simulink model "HardwareModel"  (R2023a)
settings: Solver=ode4  StartTime=0.0  StopTime=inf  FixedStep=Parameters.Simulink.time_step_s  RelTol=1e-3
undefined symbols (not defined in the file or in its folder): flight_mode, FLIGHT_MODE, joystick, Parameters, wait_time_s
libraries: px4lib x121, matrix_library x9, px4uORBlib x3, sharedutil x2, simulink_extras x1, vrlib x1
settings Model: ExtModeTrigDuration=10  Creator=thesa  LastModifiedBy=thesa
settings SolverCC: PositivePriorityOrder=on
settings OptimizationCC: EnhancedBackFolding=on  PassReuseOutputArgsAs=Individual arguments  ZeroExternalMemoryAtStartup=off  ZeroInternalMemoryAtStartup=off  MaxStackSize=64  OptimizeBlockOrder=speed  DifferentSizesBufferReuse=on  OptimizationCustomize=off  EfficientTunableParamExpr=on
settings DebuggingCC: ParameterTunabilityLossMsg=error
settings HardwareCC: ProdBitPerPointer=32  ProdBitPerSizeT=32  ProdBitPerPtrDiffT=32  ProdLargestAtomicInteger=Long  ProdLargestAtomicFloat=Double  ProdWordSize=32  ProdLongLongMode=on  ProdHWDeviceType=ARM Compatible->ARM Cortex
settings SFSimCC: SimTargetLang=C++
settings RTWCC: Description=Embedded Coder  SystemTargetFile=ert.tlc  HardwareBoard=PX4 Cube Orange  TLCOptions="-aInlineSetEventsForThisBaseRateFcn=TLC_FALSE -aSuppressMultiTaskScheduler=TLC_FALSE  -aRateBasedStepFcn=0"  TemplateMakefile=ert_default_tmf  Toolchain=GNU Tools for PX4 Autopilots  TargetLang=C++
settings CodeAppCC: ForceParamTrailComments=on  IgnoreCustomStorageClasses=off  OperatorAnnotations=on  SimulinkDataObjDesc=on  SFDataObjDesc=on  InsertBlockDesc=on
settings ERTTargetCC: SupportVariableSizeSignals=on  ExtModeTransport=3  ExtModeStaticAlloc=on  ExtModeStaticAllocSize=1024  ExtModeMexFile=ext_xcp  ExtModeIntrfLevel=Level2 - Open

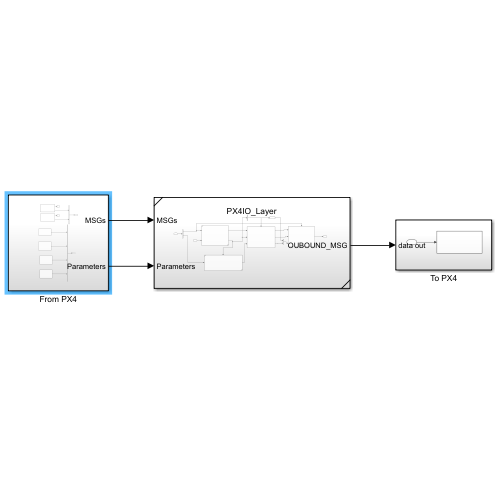
[thumbnail: Simulink's stored preview of the top-level diagram]
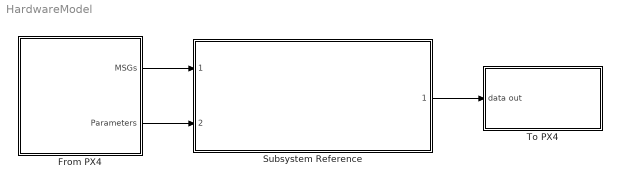
== system HardwareModel ==
  From PX4 : Subsystem
  Subsystem Reference : Subsystem  ReferencedSubsystem=PX4IO_Layer
  To PX4 : Subsystem
  wires:
  From PX4/1(MSGs) -> Subsystem Reference/1
  Subsystem Reference/1 -> To PX4/1(data out)
  From PX4/2(Parameters) -> Subsystem Reference/2

== system HardwareModel/From PX4 ==
  Bus Creator : BusCreator  Inputs=4
  Bus Creator1 : BusCreator  Inputs=2
  PX4 uORB Read : px4uORBlib/PX4 uORB Read  uORBTopic=debug_array  selectInstance=simulink_inbound  SampleTime=-1  BlockingMode=off  BlockTimeout=1e-3
  PX4 uORB Read1 : px4uORBlib/PX4 uORB Read  uORBTopic=debug_array  selectInstance=simulink_guidance  SampleTime=-1  BlockingMode=off  BlockTimeout=1e-3
  Subsystem1 : Subsystem
  Subsystem2 : Subsystem
  Subsystem3 : Subsystem
  Subsystem5 : Subsystem
  Terminator : Terminator
  Terminator1 : Terminator
  MSGs : Outport
  Parameters : Outport  Port=2
  wires:
  PX4 uORB Read/1 -> Terminator/1
  PX4 uORB Read/2 -> Bus Creator1/1  "INBOUND_MSG"
  Subsystem2/1(Control Gains) -> Bus Creator/2  "Control Gains"
  Subsystem3/1(Vehicle Parameters) -> Bus Creator/1  "Vehicle Parameters"
  Subsystem5/1(Pilot Input) -> Bus Creator/4  "Pilot Input"
  Bus Creator1/1 -> MSGs/1
  PX4 uORB Read1/1 -> Terminator1/1
  PX4 uORB Read1/2 -> Bus Creator1/2  "GUIDANCE_MSG"
  Subsystem1/1(Control Logic) -> Bus Creator/3  "Control Logic"
  Bus Creator/1 -> Parameters/1

== system HardwareModel/To PX4 ==
  data out : Inport
  PX4 uORB Write1 : px4uORBlib/PX4 uORB Write  uORBTopic=debug_array  selectInstance=simulink_outbound  MessageQueueLen=1
  wires:
  data out/1 -> PX4 uORB Write1/1

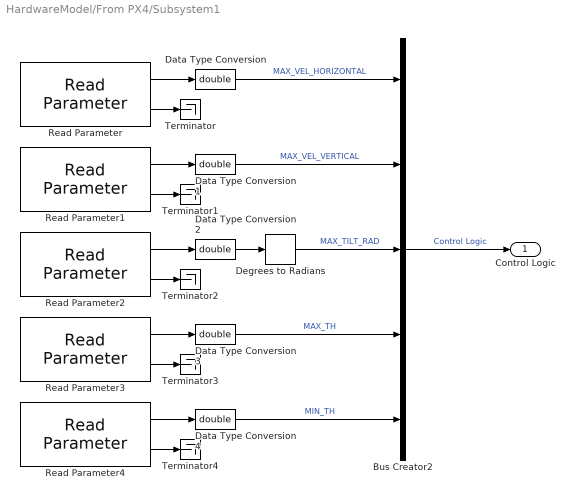
== system HardwareModel/From PX4/Subsystem1 ==
  Bus Creator2 : BusCreator  Inputs=5
  Data Type Conversion{,1..4} (5 alike) : DataTypeConversion  OutDataTypeStr=double  SaturateOnIntegerOverflow=off  RndMeth=Floor
  Degrees to Radians : simulink_extras/Transformations/Degrees to Radians
  Read Parameter : px4lib/Read Parameter  ParameterName=SM_MAX_VEL_HOR  DataType=FLOAT  SampleTime=-1
  Read Parameter1 : px4lib/Read Parameter  ParameterName=SM_MAX_VEL_VER  DataType=FLOAT  SampleTime=-1
  Read Parameter2 : px4lib/Read Parameter  ParameterName=SM_MAX_TILT  DataType=FLOAT  SampleTime=-1
  Read Parameter3 : px4lib/Read Parameter  ParameterName=SM_MAX_TH  DataType=FLOAT  SampleTime=-1
  Read Parameter4 : px4lib/Read Parameter  ParameterName=SM_MIN_TH  DataType=FLOAT  SampleTime=-1
  Terminator{,1..4} (5 alike) : Terminator
  Control Logic : Outport
  wires:
  Read Parameter4/1 -> Data Type Conversion4/1
  Read Parameter3/1 -> Data Type Conversion3/1
  Read Parameter1/1 -> Data Type Conversion1/1
  Bus Creator2/1 -> Control Logic/1  "Control Logic"
  Read Parameter/1 -> Data Type Conversion/1
  Read Parameter2/1 -> Data Type Conversion2/1
  Degrees to Radians/1 -> Bus Creator2/3  "MAX_TILT_RAD"
  Read Parameter/2 -> Terminator/1
  Read Parameter1/2 -> Terminator1/1
  Read Parameter3/2 -> Terminator3/1
  Read Parameter2/2 -> Terminator2/1
  Read Parameter4/2 -> Terminator4/1
  Data Type Conversion/1 -> Bus Creator2/1  "MAX_VEL_HORIZONTAL"
  Data Type Conversion1/1 -> Bus Creator2/2  "MAX_VEL_VERTICAL"
  Data Type Conversion2/1 -> Degrees to Radians/1
  Data Type Conversion3/1 -> Bus Creator2/4  "MAX_TH"
  Data Type Conversion4/1 -> Bus Creator2/5  "MIN_TH"

== system HardwareModel/From PX4/Subsystem2 ==
  " K-matrix control (LQR, H-inf, etc.)" : Subsystem
  Bus Creator2 : BusCreator  Inputs=9
  Subsystem : Subsystem
  Subsystem1 : Subsystem
  Subsystem2 : Subsystem
  Subsystem3 : Subsystem
  Subsystem4 : Subsystem
  Subsystem5 : Subsystem
  Subsystem6 : Subsystem
  Subsystem7 : Subsystem
  Control Gains : Outport
  wires:
  Subsystem2/1(VEL_P) -> Bus Creator2/3  "K_vel"
  Subsystem/1(POS_P) -> Bus Creator2/1  "K_pos"
  Subsystem5/1(RATE_P) -> Bus Creator2/6  "K_omega"
  Bus Creator2/1 -> Control Gains/1  "Control Gains"
  Subsystem1/1(POS_I) -> Bus Creator2/2  "K_pos_int"
  Subsystem3/1(ACC_P) -> Bus Creator2/4  "K_acc"
  Subsystem4/1(ATT_P) -> Bus Creator2/5  "K_att"
  " K-matrix control (LQR, H-inf, etc.)"/1(K_matrix_control) -> Bus Creator2/9  "K_matrix_control"
  Subsystem6/1(RATE_I) -> Bus Creator2/7  "K_omega_I"
  Subsystem7/1(RATE_D) -> Bus Creator2/8  "K_omega_dot"

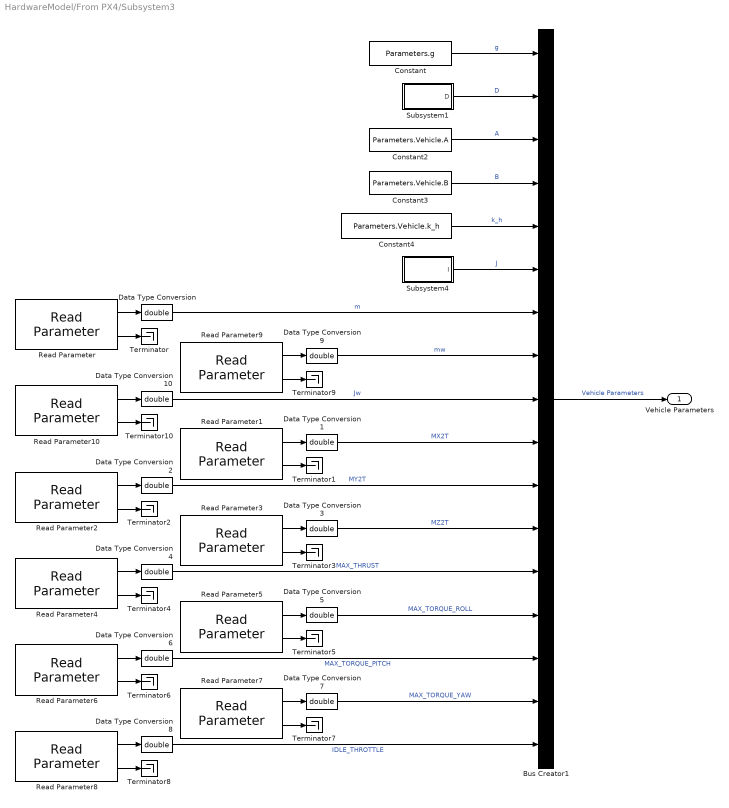
== system HardwareModel/From PX4/Subsystem3 ==
  Bus Creator1 : BusCreator  Inputs=17
  Constant : Constant  Value=Parameters.g
  Constant2 : Constant  Value=Parameters.Vehicle.A
  Constant3 : Constant  Value=Parameters.Vehicle.B
  Constant4 : Constant  Value=Parameters.Vehicle.k_h
  Data Type Conversion{,1..10} (11 alike) : DataTypeConversion  OutDataTypeStr=double  SaturateOnIntegerOverflow=off  RndMeth=Floor
  Read Parameter : px4lib/Read Parameter  ParameterName=SM_MASS  DataType=FLOAT  SampleTime=-1
  Read Parameter1 : px4lib/Read Parameter  ParameterName=SM_MX2T  DataType=FLOAT  SampleTime=-1
  Read Parameter10 : px4lib/Read Parameter  ParameterName=SM_I_ROTOR  DataType=FLOAT  SampleTime=-1
  Read Parameter2 : px4lib/Read Parameter  ParameterName=SM_MY2T  DataType=FLOAT  SampleTime=-1
  Read Parameter3 : px4lib/Read Parameter  ParameterName=SM_MZ2T  DataType=FLOAT  SampleTime=-1
  Read Parameter4 : px4lib/Read Parameter  ParameterName=SM_MAX_THRUST  DataType=FLOAT  SampleTime=-1
  Read Parameter5 : px4lib/Read Parameter  ParameterName=SM_MAX_MROLL  DataType=FLOAT  SampleTime=-1
  Read Parameter6 : px4lib/Read Parameter  ParameterName=SM_MAX_MPITCH  DataType=FLOAT  SampleTime=-1
  Read Parameter7 : px4lib/Read Parameter  ParameterName=SM_MAX_MYAW  DataType=FLOAT  SampleTime=-1
  Read Parameter8 : px4lib/Read Parameter  ParameterName=SM_IDLE_TH  DataType=FLOAT  SampleTime=-1
  Read Parameter9 : px4lib/Read Parameter  ParameterName=SM_MASS_ROTOR  DataType=FLOAT  SampleTime=-1
  Subsystem1 : Subsystem
  Subsystem4 : Subsystem
  Terminator{,1..10} (11 alike) : Terminator
  Vehicle Parameters : Outport
  wires:
  Subsystem4/1(I) -> Bus Creator1/6  "J"
  Constant3/1 -> Bus Creator1/4  "B"
  Constant/1 -> Bus Creator1/1  "g"
  Subsystem1/1(D) -> Bus Creator1/2  "D"
  Constant2/1 -> Bus Creator1/3  "A"
  Constant4/1 -> Bus Creator1/5  "k_h"
  Bus Creator1/1 -> Vehicle Parameters/1  "Vehicle Parameters"
  Data Type Conversion/1 -> Bus Creator1/7  "m"
  Data Type Conversion9/1 -> Bus Creator1/8  "mw"
  Data Type Conversion10/1 -> Bus Creator1/9  "Jw"
  Data Type Conversion1/1 -> Bus Creator1/10  "MX2T"
  Data Type Conversion2/1 -> Bus Creator1/11  "MY2T"
  Data Type Conversion3/1 -> Bus Creator1/12  "MZ2T"
  Data Type Conversion4/1 -> Bus Creator1/13  "MAX_THRUST"
  Data Type Conversion5/1 -> Bus Creator1/14  "MAX_TORQUE_ROLL"
  Data Type Conversion6/1 -> Bus Creator1/15  "MAX_TORQUE_PITCH"
  Data Type Conversion7/1 -> Bus Creator1/16  "MAX_TORQUE_YAW"
  Data Type Conversion8/1 -> Bus Creator1/17  "IDLE_THROTTLE"
  Read Parameter/2 -> Terminator/1
  Read Parameter/1 -> Data Type Conversion/1
  Read Parameter1/2 -> Terminator1/1
  Read Parameter1/1 -> Data Type Conversion1/1
  Read Parameter2/2 -> Terminator2/1
  Read Parameter2/1 -> Data Type Conversion2/1
  Read Parameter3/2 -> Terminator3/1
  Read Parameter3/1 -> Data Type Conversion3/1
  Read Parameter4/2 -> Terminator4/1
  Read Parameter4/1 -> Data Type Conversion4/1
  Read Parameter5/2 -> Terminator5/1
  Read Parameter5/1 -> Data Type Conversion5/1
  Read Parameter6/2 -> Terminator6/1
  Read Parameter6/1 -> Data Type Conversion6/1
  Read Parameter7/1 -> Data Type Conversion7/1
  Read Parameter7/2 -> Terminator7/1
  Read Parameter8/1 -> Data Type Conversion8/1
  Read Parameter8/2 -> Terminator8/1
  Read Parameter9/1 -> Data Type Conversion9/1
  Read Parameter9/2 -> Terminator9/1
  Read Parameter10/1 -> Data Type Conversion10/1
  Read Parameter10/2 -> Terminator10/1

== system HardwareModel/From PX4/Subsystem5 ==
  Bus Creator4 : BusCreator  Inputs=4
  Subsystem : Subsystem
  Subsystem1 : Subsystem
  Pilot Input : Outport
  wires:
  Subsystem/1(sticks) -> Bus Creator4/1  "Sticks"
  Bus Creator4/1 -> Pilot Input/1  "Pilot Input"
  Subsystem1/1(Parameters) -> Bus Creator4/4  "Parameters"
  Subsystem/2(FLIGHT_MODE) -> Bus Creator4/2  "FLIGHT_MODE"
  Subsystem/3(ARMED) -> Bus Creator4/3  "ARMED"

== system HardwareModel/From PX4/Subsystem2/ K-matrix control (LQR, H-inf, etc.) ==
  Bus Creator : BusCreator  Inputs=3
  Data Type Conversion9 : DataTypeConversion  OutDataTypeStr=boolean  SaturateOnIntegerOverflow=off  RndMeth=Floor
  Read Parameter9 : px4lib/Read Parameter  ParameterName=SM_EN_K_CONROL  DataType=INT32  SampleTime=-1
  Subsystem5 : Subsystem
  Subsystem6 : Subsystem
  Terminator9 : Terminator
  K_matrix_control : Outport
  wires:
  Bus Creator/1 -> K_matrix_control/1  "K_matrix_control"
  Subsystem6/1(K_matrix) -> Bus Creator/2  "K"
  Data Type Conversion9/1 -> Bus Creator/1  "EN"
  Subsystem5/1(K_pos_int) -> Bus Creator/3  "K_pos_int"
  Read Parameter9/2 -> Terminator9/1
  Read Parameter9/1 -> Data Type Conversion9/1

== system HardwareModel/From PX4/Subsystem2/Subsystem ==
  Create Diagonal Matrix : matrix_library/Create Diagonal Matrix
      settings: LibrarySourceBlock=|
      | simulink/Matrix
      | Operations/Create Diagonal
      | Matrix
  Data Type Conversion : DataTypeConversion  OutDataTypeStr=double  SaturateOnIntegerOverflow=off  RndMeth=Floor
  Mux : Mux  Inputs=3
  Read Parameter : px4lib/Read Parameter  ParameterName=SM_POS_P1  DataType=FLOAT  SampleTime=-1
  Read Parameter1 : px4lib/Read Parameter  ParameterName=SM_POS_P2  DataType=FLOAT  SampleTime=-1
  Read Parameter2 : px4lib/Read Parameter  ParameterName=SM_POS_P3  DataType=FLOAT  SampleTime=-1
  Terminator : Terminator
  Terminator1 : Terminator
  Terminator2 : Terminator
  POS_P : Outport
  wires:
  Read Parameter2/1 -> Mux/3
  Data Type Conversion/1 -> Create Diagonal Matrix/1
  Read Parameter2/2 -> Terminator2/1
  Read Parameter1/2 -> Terminator1/1
  Read Parameter/2 -> Terminator/1
  Read Parameter1/1 -> Mux/2
  Mux/1 -> Data Type Conversion/1
  Read Parameter/1 -> Mux/1
  Create Diagonal Matrix/1 -> POS_P/1

== system HardwareModel/From PX4/Subsystem2/Subsystem1 ==
  Create Diagonal Matrix : matrix_library/Create Diagonal Matrix
      settings: LibrarySourceBlock=|
      | simulink/Matrix
      | Operations/Create Diagonal
      | Matrix
  Data Type Conversion : DataTypeConversion  OutDataTypeStr=double  SaturateOnIntegerOverflow=off  RndMeth=Floor
  Mux : Mux  Inputs=3
  Read Parameter : px4lib/Read Parameter  ParameterName=SM_POS_I1  DataType=FLOAT  SampleTime=-1
  Read Parameter1 : px4lib/Read Parameter  ParameterName=SM_POS_I2  DataType=FLOAT  SampleTime=-1
  Read Parameter2 : px4lib/Read Parameter  ParameterName=SM_POS_I3  DataType=FLOAT  SampleTime=-1
  Terminator : Terminator
  Terminator1 : Terminator
  Terminator2 : Terminator
  POS_I : Outport
  wires:
  Read Parameter2/1 -> Mux/3
  Data Type Conversion/1 -> Create Diagonal Matrix/1
  Read Parameter2/2 -> Terminator2/1
  Read Parameter1/2 -> Terminator1/1
  Read Parameter/2 -> Terminator/1
  Read Parameter1/1 -> Mux/2
  Mux/1 -> Data Type Conversion/1
  Read Parameter/1 -> Mux/1
  Create Diagonal Matrix/1 -> POS_I/1

== system HardwareModel/From PX4/Subsystem2/Subsystem2 ==
  Create Diagonal Matrix : matrix_library/Create Diagonal Matrix
      settings: LibrarySourceBlock=|
      | simulink/Matrix
      | Operations/Create Diagonal
      | Matrix
  Data Type Conversion : DataTypeConversion  OutDataTypeStr=double  SaturateOnIntegerOverflow=off  RndMeth=Floor
  Mux : Mux  Inputs=3
  Read Parameter : px4lib/Read Parameter  ParameterName=SM_VEL_P1  DataType=FLOAT  SampleTime=-1
  Read Parameter1 : px4lib/Read Parameter  ParameterName=SM_VEL_P2  DataType=FLOAT  SampleTime=-1
  Read Parameter2 : px4lib/Read Parameter  ParameterName=SM_VEL_P3  DataType=FLOAT  SampleTime=-1
  Terminator : Terminator
  Terminator1 : Terminator
  Terminator2 : Terminator
  VEL_P : Outport
  wires:
  Read Parameter2/1 -> Mux/3
  Data Type Conversion/1 -> Create Diagonal Matrix/1
  Read Parameter2/2 -> Terminator2/1
  Read Parameter1/2 -> Terminator1/1
  Read Parameter/2 -> Terminator/1
  Read Parameter1/1 -> Mux/2
  Mux/1 -> Data Type Conversion/1
  Read Parameter/1 -> Mux/1
  Create Diagonal Matrix/1 -> VEL_P/1

== system HardwareModel/From PX4/Subsystem2/Subsystem3 ==
  Create Diagonal Matrix : matrix_library/Create Diagonal Matrix
      settings: LibrarySourceBlock=|
      | simulink/Matrix
      | Operations/Create Diagonal
      | Matrix
  Data Type Conversion : DataTypeConversion  OutDataTypeStr=double  SaturateOnIntegerOverflow=off  RndMeth=Floor
  Mux : Mux  Inputs=3
  Read Parameter : px4lib/Read Parameter  ParameterName=SM_ACC_P1  DataType=FLOAT  SampleTime=-1
  Read Parameter1 : px4lib/Read Parameter  ParameterName=SM_ACC_P2  DataType=FLOAT  SampleTime=-1
  Read Parameter2 : px4lib/Read Parameter  ParameterName=SM_ACC_P3  DataType=FLOAT  SampleTime=-1
  Terminator : Terminator
  Terminator1 : Terminator
  Terminator2 : Terminator
  ACC_P : Outport
  wires:
  Read Parameter2/1 -> Mux/3
  Data Type Conversion/1 -> Create Diagonal Matrix/1
  Read Parameter2/2 -> Terminator2/1
  Read Parameter1/2 -> Terminator1/1
  Read Parameter/2 -> Terminator/1
  Read Parameter1/1 -> Mux/2
  Mux/1 -> Data Type Conversion/1
  Read Parameter/1 -> Mux/1
  Create Diagonal Matrix/1 -> ACC_P/1

== system HardwareModel/From PX4/Subsystem2/Subsystem4 ==
  Create Diagonal Matrix : matrix_library/Create Diagonal Matrix
      settings: LibrarySourceBlock=|
      | simulink/Matrix
      | Operations/Create Diagonal
      | Matrix
  Data Type Conversion : DataTypeConversion  OutDataTypeStr=double  SaturateOnIntegerOverflow=off  RndMeth=Floor
  Mux : Mux  Inputs=3
  Read Parameter : px4lib/Read Parameter  ParameterName=SM_ATT_P1  DataType=FLOAT  SampleTime=-1
  Read Parameter1 : px4lib/Read Parameter  ParameterName=SM_ATT_P2  DataType=FLOAT  SampleTime=-1
  Read Parameter2 : px4lib/Read Parameter  ParameterName=SM_ATT_P3  DataType=FLOAT  SampleTime=-1
  Terminator : Terminator
  Terminator1 : Terminator
  Terminator2 : Terminator
  ATT_P : Outport
  wires:
  Read Parameter2/1 -> Mux/3
  Data Type Conversion/1 -> Create Diagonal Matrix/1
  Read Parameter2/2 -> Terminator2/1
  Read Parameter1/2 -> Terminator1/1
  Read Parameter/2 -> Terminator/1
  Read Parameter1/1 -> Mux/2
  Mux/1 -> Data Type Conversion/1
  Read Parameter/1 -> Mux/1
  Create Diagonal Matrix/1 -> ATT_P/1

== system HardwareModel/From PX4/Subsystem2/Subsystem5 ==
  Create Diagonal Matrix : matrix_library/Create Diagonal Matrix
      settings: LibrarySourceBlock=|
      | simulink/Matrix
      | Operations/Create Diagonal
      | Matrix
  Data Type Conversion : DataTypeConversion  OutDataTypeStr=double  SaturateOnIntegerOverflow=off  RndMeth=Floor
  Mux : Mux  Inputs=3
  Read Parameter : px4lib/Read Parameter  ParameterName=SM_RATE_P1  DataType=FLOAT  SampleTime=-1
  Read Parameter1 : px4lib/Read Parameter  ParameterName=SM_RATE_P2  DataType=FLOAT  SampleTime=-1
  Read Parameter2 : px4lib/Read Parameter  ParameterName=SM_RATE_P3  DataType=FLOAT  SampleTime=-1
  Terminator : Terminator
  Terminator1 : Terminator
  Terminator2 : Terminator
  RATE_P : Outport
  wires:
  Read Parameter2/1 -> Mux/3
  Data Type Conversion/1 -> Create Diagonal Matrix/1
  Read Parameter2/2 -> Terminator2/1
  Read Parameter1/2 -> Terminator1/1
  Read Parameter/2 -> Terminator/1
  Read Parameter1/1 -> Mux/2
  Mux/1 -> Data Type Conversion/1
  Read Parameter/1 -> Mux/1
  Create Diagonal Matrix/1 -> RATE_P/1

== system HardwareModel/From PX4/Subsystem2/Subsystem6 ==
  Create Diagonal Matrix : matrix_library/Create Diagonal Matrix
      settings: LibrarySourceBlock=|
      | simulink/Matrix
      | Operations/Create Diagonal
      | Matrix
  Data Type Conversion : DataTypeConversion  OutDataTypeStr=double  SaturateOnIntegerOverflow=off  RndMeth=Floor
  Mux : Mux  Inputs=3
  Read Parameter : px4lib/Read Parameter  ParameterName=SM_RATE_I1  DataType=FLOAT  SampleTime=-1
  Read Parameter1 : px4lib/Read Parameter  ParameterName=SM_RATE_I2  DataType=FLOAT  SampleTime=-1
  Read Parameter2 : px4lib/Read Parameter  ParameterName=SM_RATE_I3  DataType=FLOAT  SampleTime=-1
  Terminator : Terminator
  Terminator1 : Terminator
  Terminator2 : Terminator
  RATE_I : Outport
  wires:
  Create Diagonal Matrix/1 -> RATE_I/1
  Read Parameter/1 -> Mux/1
  Mux/1 -> Data Type Conversion/1
  Read Parameter1/1 -> Mux/2
  Read Parameter/2 -> Terminator/1
  Read Parameter1/2 -> Terminator1/1
  Read Parameter2/2 -> Terminator2/1
  Data Type Conversion/1 -> Create Diagonal Matrix/1
  Read Parameter2/1 -> Mux/3

== system HardwareModel/From PX4/Subsystem2/Subsystem7 ==
  Create Diagonal Matrix : matrix_library/Create Diagonal Matrix
      settings: LibrarySourceBlock=|
      | simulink/Matrix
      | Operations/Create Diagonal
      | Matrix
  Data Type Conversion : DataTypeConversion  OutDataTypeStr=double  SaturateOnIntegerOverflow=off  RndMeth=Floor
  Mux : Mux  Inputs=3
  Read Parameter : px4lib/Read Parameter  ParameterName=SM_RATE_D1  DataType=FLOAT  SampleTime=-1
  Read Parameter1 : px4lib/Read Parameter  ParameterName=SM_RATE_D2  DataType=FLOAT  SampleTime=-1
  Read Parameter2 : px4lib/Read Parameter  ParameterName=SM_RATE_D3  DataType=FLOAT  SampleTime=-1
  Terminator : Terminator
  Terminator1 : Terminator
  Terminator2 : Terminator
  RATE_D : Outport
  wires:
  Create Diagonal Matrix/1 -> RATE_D/1
  Read Parameter/1 -> Mux/1
  Mux/1 -> Data Type Conversion/1
  Read Parameter1/1 -> Mux/2
  Read Parameter/2 -> Terminator/1
  Read Parameter1/2 -> Terminator1/1
  Read Parameter2/2 -> Terminator2/1
  Data Type Conversion/1 -> Create Diagonal Matrix/1
  Read Parameter2/1 -> Mux/3

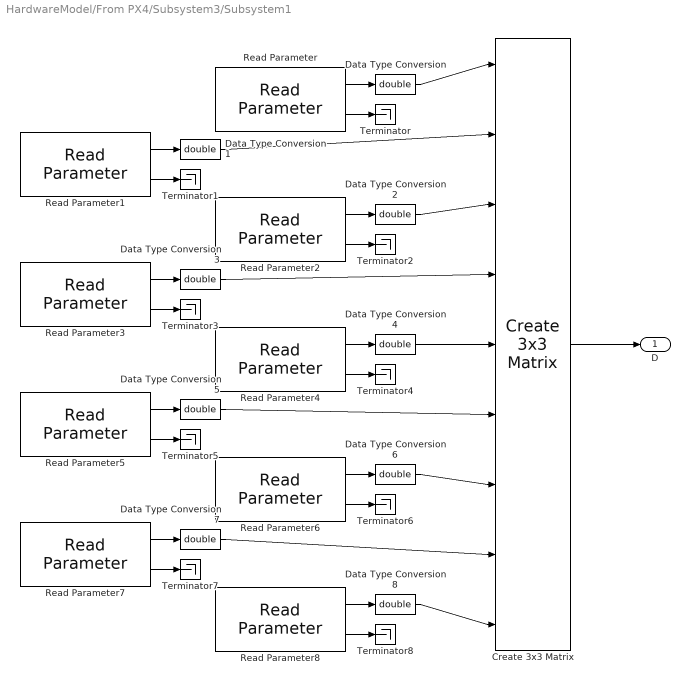
== system HardwareModel/From PX4/Subsystem3/Subsystem1 ==
  Create 3x3 Matrix : sharedutil/Create 3x3 Matrix  aMode=aMode
      settings: LibrarySourceBlock=aerolibutil/Create 3x3 Matrix
  Data Type Conversion{,1..8} (9 alike) : DataTypeConversion  OutDataTypeStr=double  SaturateOnIntegerOverflow=off  RndMeth=Floor
  Read Parameter : px4lib/Read Parameter  ParameterName=SM_D11  DataType=FLOAT  SampleTime=-1
  Read Parameter1 : px4lib/Read Parameter  ParameterName=SM_D12  DataType=FLOAT  SampleTime=-1
  Read Parameter2 : px4lib/Read Parameter  ParameterName=SM_D13  DataType=FLOAT  SampleTime=-1
  Read Parameter3 : px4lib/Read Parameter  ParameterName=SM_D21  DataType=FLOAT  SampleTime=-1
  Read Parameter4 : px4lib/Read Parameter  ParameterName=SM_D22  DataType=FLOAT  SampleTime=-1
  Read Parameter5 : px4lib/Read Parameter  ParameterName=SM_D23  DataType=FLOAT  SampleTime=-1
  Read Parameter6 : px4lib/Read Parameter  ParameterName=SM_D31  DataType=FLOAT  SampleTime=-1
  Read Parameter7 : px4lib/Read Parameter  ParameterName=SM_D32  DataType=FLOAT  SampleTime=-1
  Read Parameter8 : px4lib/Read Parameter  ParameterName=SM_D33  DataType=FLOAT  SampleTime=-1
  Terminator{,1..8} (9 alike) : Terminator
  D : Outport
  wires:
  Read Parameter/2 -> Terminator/1
  Read Parameter/1 -> Data Type Conversion/1
  Create 3x3 Matrix/1 -> D/1
  Data Type Conversion/1 -> Create 3x3 Matrix/1
  Read Parameter1/1 -> Data Type Conversion1/1
  Read Parameter1/2 -> Terminator1/1
  Data Type Conversion1/1 -> Create 3x3 Matrix/2
  Read Parameter2/1 -> Data Type Conversion2/1
  Read Parameter2/2 -> Terminator2/1
  Data Type Conversion2/1 -> Create 3x3 Matrix/3
  Read Parameter3/1 -> Data Type Conversion3/1
  Read Parameter3/2 -> Terminator3/1
  Data Type Conversion3/1 -> Create 3x3 Matrix/4
  Read Parameter4/1 -> Data Type Conversion4/1
  Read Parameter4/2 -> Terminator4/1
  Data Type Conversion4/1 -> Create 3x3 Matrix/5
  Read Parameter5/1 -> Data Type Conversion5/1
  Read Parameter5/2 -> Terminator5/1
  Data Type Conversion5/1 -> Create 3x3 Matrix/6
  Read Parameter6/1 -> Data Type Conversion6/1
  Read Parameter6/2 -> Terminator6/1
  Data Type Conversion6/1 -> Create 3x3 Matrix/7
  Read Parameter7/1 -> Data Type Conversion7/1
  Read Parameter7/2 -> Terminator7/1
  Data Type Conversion7/1 -> Create 3x3 Matrix/8
  Read Parameter8/1 -> Data Type Conversion8/1
  Read Parameter8/2 -> Terminator8/1
  Data Type Conversion8/1 -> Create 3x3 Matrix/9

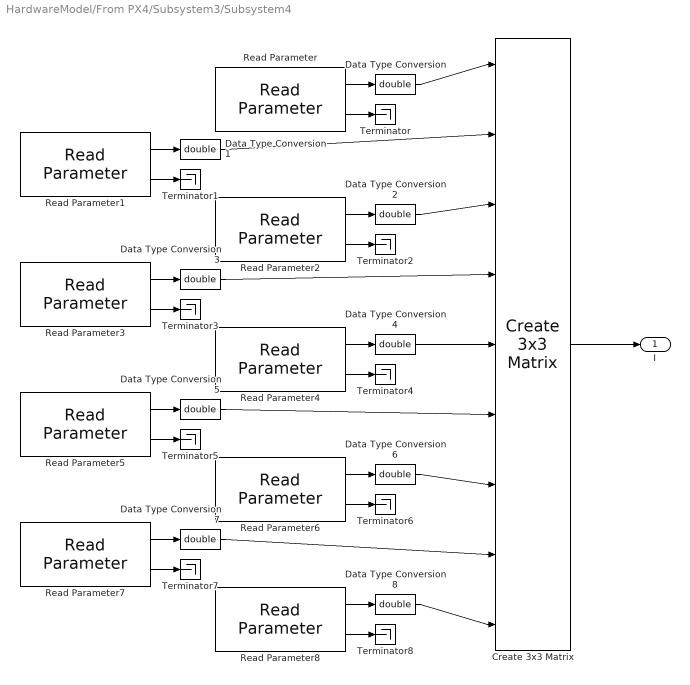
== system HardwareModel/From PX4/Subsystem3/Subsystem4 ==
  Create 3x3 Matrix : sharedutil/Create 3x3 Matrix  aMode=aMode
      settings: LibrarySourceBlock=aerolibutil/Create 3x3 Matrix
  Data Type Conversion{,1..8} (9 alike) : DataTypeConversion  OutDataTypeStr=double  SaturateOnIntegerOverflow=off  RndMeth=Floor
  Read Parameter : px4lib/Read Parameter  ParameterName=SM_I11  DataType=FLOAT  SampleTime=-1
  Read Parameter1 : px4lib/Read Parameter  ParameterName=SM_I12  DataType=FLOAT  SampleTime=-1
  Read Parameter2 : px4lib/Read Parameter  ParameterName=SM_I13  DataType=FLOAT  SampleTime=-1
  Read Parameter3 : px4lib/Read Parameter  ParameterName=SM_I21  DataType=FLOAT  SampleTime=-1
  Read Parameter4 : px4lib/Read Parameter  ParameterName=SM_I22  DataType=FLOAT  SampleTime=-1
  Read Parameter5 : px4lib/Read Parameter  ParameterName=SM_I23  DataType=FLOAT  SampleTime=-1
  Read Parameter6 : px4lib/Read Parameter  ParameterName=SM_I31  DataType=FLOAT  SampleTime=-1
  Read Parameter7 : px4lib/Read Parameter  ParameterName=SM_I32  DataType=FLOAT  SampleTime=-1
  Read Parameter8 : px4lib/Read Parameter  ParameterName=SM_I33  DataType=FLOAT  SampleTime=-1
  Terminator{,1..8} (9 alike) : Terminator
  I : Outport
  wires:
  Read Parameter/2 -> Terminator/1
  Read Parameter/1 -> Data Type Conversion/1
  Create 3x3 Matrix/1 -> I/1
  Data Type Conversion/1 -> Create 3x3 Matrix/1
  Read Parameter1/1 -> Data Type Conversion1/1
  Read Parameter1/2 -> Terminator1/1
  Data Type Conversion1/1 -> Create 3x3 Matrix/2
  Read Parameter2/1 -> Data Type Conversion2/1
  Read Parameter2/2 -> Terminator2/1
  Data Type Conversion2/1 -> Create 3x3 Matrix/3
  Read Parameter3/1 -> Data Type Conversion3/1
  Read Parameter3/2 -> Terminator3/1
  Data Type Conversion3/1 -> Create 3x3 Matrix/4
  Read Parameter4/1 -> Data Type Conversion4/1
  Read Parameter4/2 -> Terminator4/1
  Data Type Conversion4/1 -> Create 3x3 Matrix/5
  Read Parameter5/1 -> Data Type Conversion5/1
  Read Parameter5/2 -> Terminator5/1
  Data Type Conversion5/1 -> Create 3x3 Matrix/6
  Read Parameter6/1 -> Data Type Conversion6/1
  Read Parameter6/2 -> Terminator6/1
  Data Type Conversion6/1 -> Create 3x3 Matrix/7
  Read Parameter7/1 -> Data Type Conversion7/1
  Read Parameter7/2 -> Terminator7/1
  Data Type Conversion7/1 -> Create 3x3 Matrix/8
  Read Parameter8/1 -> Data Type Conversion8/1
  Read Parameter8/2 -> Terminator8/1
  Data Type Conversion8/1 -> Create 3x3 Matrix/9

== system HardwareModel/From PX4/Subsystem5/Subsystem ==
  Bus Creator4 : BusCreator  Inputs=4
  Subsystem1 : Subsystem  Variant=on  VariantControlMode=label  VariantControl=Choice  LabelModeActiveChoice=Choice_1
  sticks : Outport
  FLIGHT_MODE : Outport  Port=2
  ARMED : Outport  Port=3
  wires:
  Bus Creator4/1 -> sticks/1
  Subsystem1/1(roll_stick) -> Bus Creator4/1
  Subsystem1/2(pitch_stick) -> Bus Creator4/2
  Subsystem1/3(yaw_stick) -> Bus Creator4/3
  Subsystem1/4(Throttle_stick) -> Bus Creator4/4
  Subsystem1/5(FLIGHT_MODE) -> FLIGHT_MODE/1
  Subsystem1/6(ARMED) -> ARMED/1

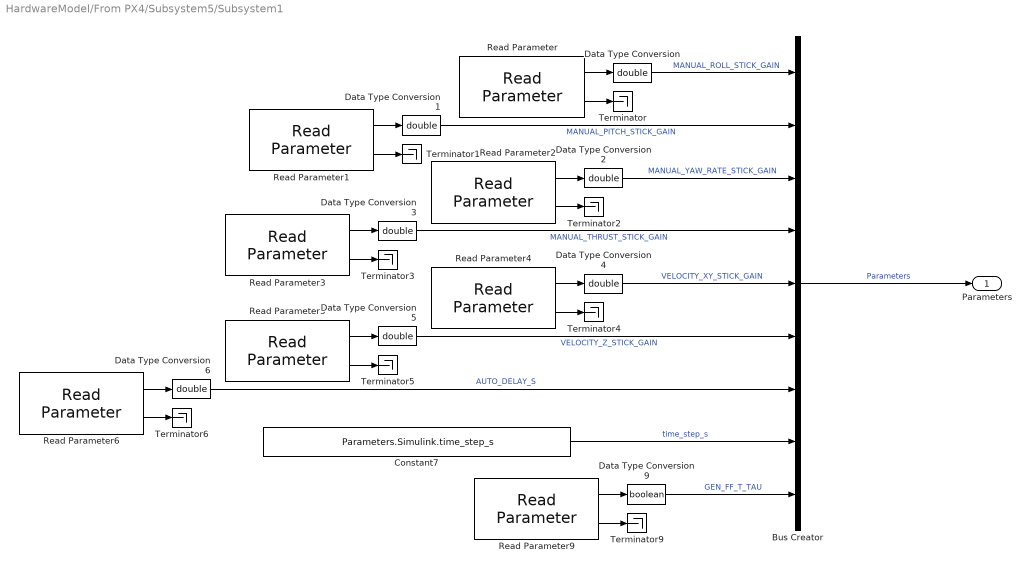
== system HardwareModel/From PX4/Subsystem5/Subsystem1 ==
  Bus Creator : BusCreator  Inputs=9
  Constant7 : Constant  Value=Parameters.Simulink.time_step_s
  Data Type Conversion{,1..6} (7 alike) : DataTypeConversion  OutDataTypeStr=double  SaturateOnIntegerOverflow=off  RndMeth=Floor
  Data Type Conversion9 : DataTypeConversion  OutDataTypeStr=boolean  SaturateOnIntegerOverflow=off  RndMeth=Floor
  Read Parameter : px4lib/Read Parameter  ParameterName=SM_ROLL_SGAIN  DataType=FLOAT  SampleTime=-1
  Read Parameter1 : px4lib/Read Parameter  ParameterName=SM_PITCH_SGAIN  DataType=FLOAT  SampleTime=-1
  Read Parameter2 : px4lib/Read Parameter  ParameterName=SM_YAWR_SGAIN  DataType=FLOAT  SampleTime=-1
  Read Parameter3 : px4lib/Read Parameter  ParameterName=SM_THRUST_SGAIN  DataType=FLOAT  SampleTime=-1
  Read Parameter4 : px4lib/Read Parameter  ParameterName=SM_VXY_SGAIN  DataType=FLOAT  SampleTime=-1
  Read Parameter5 : px4lib/Read Parameter  ParameterName=SM_VZ_SGAIN  DataType=FLOAT  SampleTime=-1
  Read Parameter6 : px4lib/Read Parameter  ParameterName=SM_AUTO_DELAY_S  DataType=FLOAT  SampleTime=-1
  Read Parameter9 : px4lib/Read Parameter  ParameterName=SM_EN_FF_T_TAU  DataType=INT32  SampleTime=-1
  Terminator{,1..6,9} (8 alike) : Terminator
  Parameters : Outport
  wires:
  Data Type Conversion/1 -> Bus Creator/1  "MANUAL_ROLL_STICK_GAIN"
  Bus Creator/1 -> Parameters/1  "Parameters"
  Data Type Conversion1/1 -> Bus Creator/2  "MANUAL_PITCH_STICK_GAIN"
  Data Type Conversion2/1 -> Bus Creator/3  "MANUAL_YAW_RATE_STICK_GAIN"
  Data Type Conversion3/1 -> Bus Creator/4  "MANUAL_THRUST_STICK_GAIN"
  Data Type Conversion4/1 -> Bus Creator/5  "VELOCITY_XY_STICK_GAIN"
  Data Type Conversion5/1 -> Bus Creator/6  "VELOCITY_Z_STICK_GAIN"
  Data Type Conversion6/1 -> Bus Creator/7  "AUTO_DELAY_S"
  Constant7/1 -> Bus Creator/8  "time_step_s"
  Read Parameter/1 -> Data Type Conversion/1
  Read Parameter/2 -> Terminator/1
  Read Parameter1/1 -> Data Type Conversion1/1
  Read Parameter1/2 -> Terminator1/1
  Read Parameter2/2 -> Terminator2/1
  Read Parameter2/1 -> Data Type Conversion2/1
  Read Parameter3/2 -> Terminator3/1
  Read Parameter3/1 -> Data Type Conversion3/1
  Read Parameter4/2 -> Terminator4/1
  Read Parameter4/1 -> Data Type Conversion4/1
  Read Parameter5/2 -> Terminator5/1
  Read Parameter5/1 -> Data Type Conversion5/1
  Read Parameter6/2 -> Terminator6/1
  Read Parameter6/1 -> Data Type Conversion6/1
  Read Parameter9/1 -> Data Type Conversion9/1
  Read Parameter9/2 -> Terminator9/1
  Data Type Conversion9/1 -> Bus Creator/9  "GEN_FF_T_TAU"

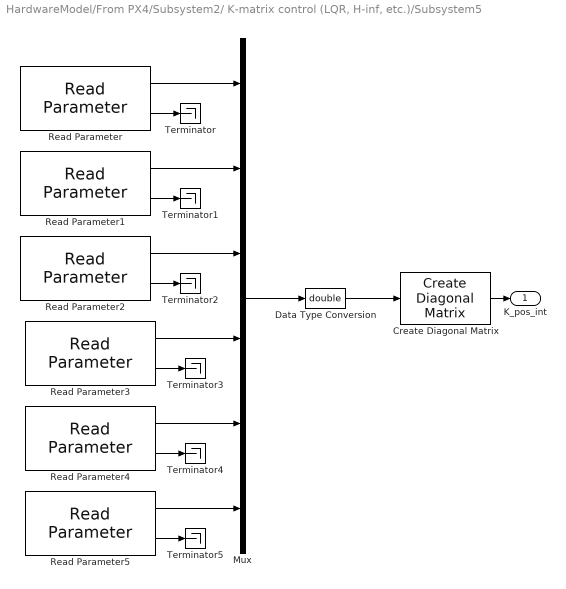
== system HardwareModel/From PX4/Subsystem2/ K-matrix control (LQR, H-inf, etc.)/Subsystem5 ==
  Create Diagonal Matrix : matrix_library/Create Diagonal Matrix
      settings: LibrarySourceBlock=|
      | simulink/Matrix
      | Operations/Create Diagonal
      | Matrix
  Data Type Conversion : DataTypeConversion  OutDataTypeStr=double  SaturateOnIntegerOverflow=off  RndMeth=Floor
  Mux : Mux  Inputs=6
  Read Parameter : px4lib/Read Parameter  ParameterName=SM_POS_K_I_1  DataType=FLOAT  SampleTime=-1
  Read Parameter1 : px4lib/Read Parameter  ParameterName=SM_POS_K_I_2  DataType=FLOAT  SampleTime=-1
  Read Parameter2 : px4lib/Read Parameter  ParameterName=SM_POS_K_I_3  DataType=FLOAT  SampleTime=-1
  Read Parameter3 : px4lib/Read Parameter  ParameterName=SM_POS_K_I_4  DataType=FLOAT  SampleTime=-1
  Read Parameter4 : px4lib/Read Parameter  ParameterName=SM_POS_K_I_5  DataType=FLOAT  SampleTime=-1
  Read Parameter5 : px4lib/Read Parameter  ParameterName=SM_POS_K_I_6  DataType=FLOAT  SampleTime=-1
  Terminator{,1..5} (6 alike) : Terminator
  K_pos_int : Outport
  wires:
  Read Parameter2/1 -> Mux/3
  Data Type Conversion/1 -> Create Diagonal Matrix/1
  Read Parameter2/2 -> Terminator2/1
  Read Parameter1/2 -> Terminator1/1
  Read Parameter/2 -> Terminator/1
  Read Parameter1/1 -> Mux/2
  Mux/1 -> Data Type Conversion/1
  Read Parameter/1 -> Mux/1
  Create Diagonal Matrix/1 -> K_pos_int/1
  Read Parameter3/1 -> Mux/4
  Read Parameter5/1 -> Mux/6
  Read Parameter3/2 -> Terminator3/1
  Read Parameter5/2 -> Terminator5/1
  Read Parameter4/2 -> Terminator4/1
  Read Parameter4/1 -> Mux/5

== system HardwareModel/From PX4/Subsystem2/ K-matrix control (LQR, H-inf, etc.)/Subsystem6 ==
  Matrix Concatenate : Concatenate  NumInputs=4  Mode=Multidimensional array
  Subsystem : Subsystem
  Subsystem1 : Subsystem
  Subsystem2 : Subsystem
  Subsystem3 : Subsystem
  K_matrix : Outport
  wires:
  Matrix Concatenate/1 -> K_matrix/1
  Subsystem/1(K_(1,:)) -> Matrix Concatenate/1
  Subsystem1/1(K_(2,:)) -> Matrix Concatenate/2
  Subsystem2/1(K_(3,:)) -> Matrix Concatenate/3
  Subsystem3/1(K_(4,:)) -> Matrix Concatenate/4

== system HardwareModel/From PX4/Subsystem5/Subsystem/Subsystem1 ==
  Disabled : Subsystem  VariantControl=Choice_1
  Joytick : Subsystem  VariantControl=Choice
  Sliders : Subsystem  VariantControl=Choice_2
  roll_stick : Outport
  pitch_stick : Outport  Port=2
  yaw_stick : Outport  Port=3
  Throttle_stick : Outport  Port=4
  FLIGHT_MODE : Outport  Port=5
  ARMED : Outport  Port=6

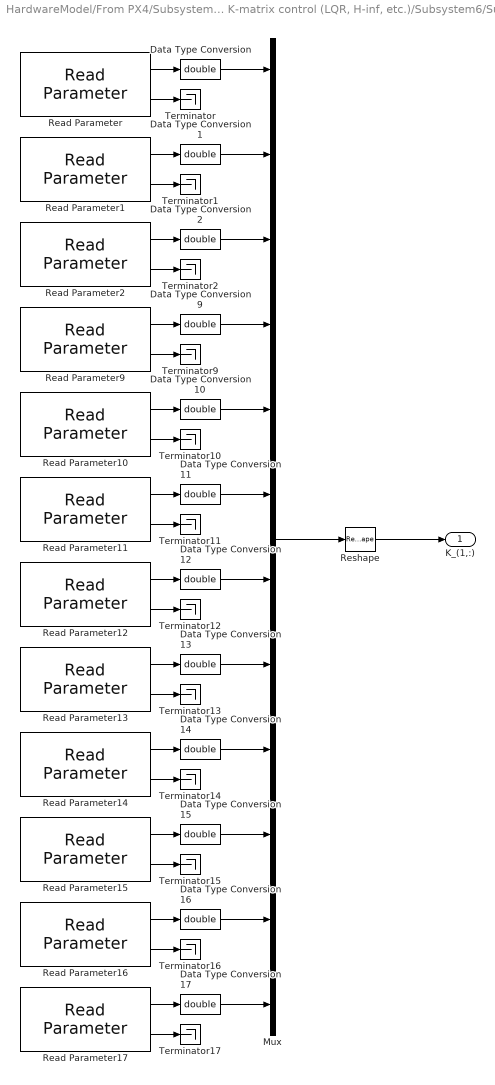
== system HardwareModel/From PX4/Subsystem2/ K-matrix control (LQR, H-inf, etc.)/Subsystem6/Subsystem ==
  Data Type Conversion{,1..2,9..17} (12 alike) : DataTypeConversion  OutDataTypeStr=double  SaturateOnIntegerOverflow=off  RndMeth=Floor
  Mux : Mux  Inputs=12
  Read Parameter : px4lib/Read Parameter  ParameterName=SM_K_1_1  DataType=FLOAT  SampleTime=-1
  Read Parameter1 : px4lib/Read Parameter  ParameterName=SM_K_1_2  DataType=FLOAT  SampleTime=-1
  Read Parameter10 : px4lib/Read Parameter  ParameterName=SM_K_1_5  DataType=FLOAT  SampleTime=-1
  Read Parameter11 : px4lib/Read Parameter  ParameterName=SM_K_1_6  DataType=FLOAT  SampleTime=-1
  Read Parameter12 : px4lib/Read Parameter  ParameterName=SM_K_1_7  DataType=FLOAT  SampleTime=-1
  Read Parameter13 : px4lib/Read Parameter  ParameterName=SM_K_1_8  DataType=FLOAT  SampleTime=-1
  Read Parameter14 : px4lib/Read Parameter  ParameterName=SM_K_1_9  DataType=FLOAT  SampleTime=-1
  Read Parameter15 : px4lib/Read Parameter  ParameterName=SM_K_1_10  DataType=FLOAT  SampleTime=-1
  Read Parameter16 : px4lib/Read Parameter  ParameterName=SM_K_1_11  DataType=FLOAT  SampleTime=-1
  Read Parameter17 : px4lib/Read Parameter  ParameterName=SM_K_1_12  DataType=FLOAT  SampleTime=-1
  Read Parameter2 : px4lib/Read Parameter  ParameterName=SM_K_1_3  DataType=FLOAT  SampleTime=-1
  Read Parameter9 : px4lib/Read Parameter  ParameterName=SM_K_1_4  DataType=FLOAT  SampleTime=-1
  Reshape : Reshape  OutputDimensionality=Row vector (2-D)
  Terminator{,1..2,9..17} (12 alike) : Terminator
  K_(1,:) : Outport
  wires:
  Read Parameter15/2 -> Terminator15/1
  Read Parameter9/2 -> Terminator9/1
  Read Parameter17/2 -> Terminator17/1
  Data Type Conversion10/1 -> Mux/5
  Read Parameter12/2 -> Terminator12/1
  Read Parameter14/2 -> Terminator14/1
  Read Parameter14/1 -> Data Type Conversion14/1
  Read Parameter2/2 -> Terminator2/1
  Read Parameter15/1 -> Data Type Conversion15/1
  Data Type Conversion/1 -> Mux/1
  Data Type Conversion11/1 -> Mux/6
  Data Type Conversion17/1 -> Mux/12
  Read Parameter11/1 -> Data Type Conversion11/1
  Data Type Conversion16/1 -> Mux/11
  Read Parameter10/1 -> Data Type Conversion10/1
  Read Parameter17/1 -> Data Type Conversion17/1
  Read Parameter10/2 -> Terminator10/1
  Data Type Conversion15/1 -> Mux/10
  Read Parameter/2 -> Terminator/1
  Data Type Conversion13/1 -> Mux/8
  Read Parameter9/1 -> Data Type Conversion9/1
  Read Parameter/1 -> Data Type Conversion/1
  Read Parameter1/1 -> Data Type Conversion1/1
  Read Parameter13/2 -> Terminator13/1
  Read Parameter1/2 -> Terminator1/1
  Data Type Conversion12/1 -> Mux/7
  Read Parameter11/2 -> Terminator11/1
  Read Parameter2/1 -> Data Type Conversion2/1
  Data Type Conversion2/1 -> Mux/3
  Read Parameter12/1 -> Data Type Conversion12/1
  Read Parameter13/1 -> Data Type Conversion13/1
  Data Type Conversion9/1 -> Mux/4
  Data Type Conversion14/1 -> Mux/9
  Read Parameter16/2 -> Terminator16/1
  Data Type Conversion1/1 -> Mux/2
  Read Parameter16/1 -> Data Type Conversion16/1
  Mux/1 -> Reshape/1
  Reshape/1 -> K_(1,:)/1

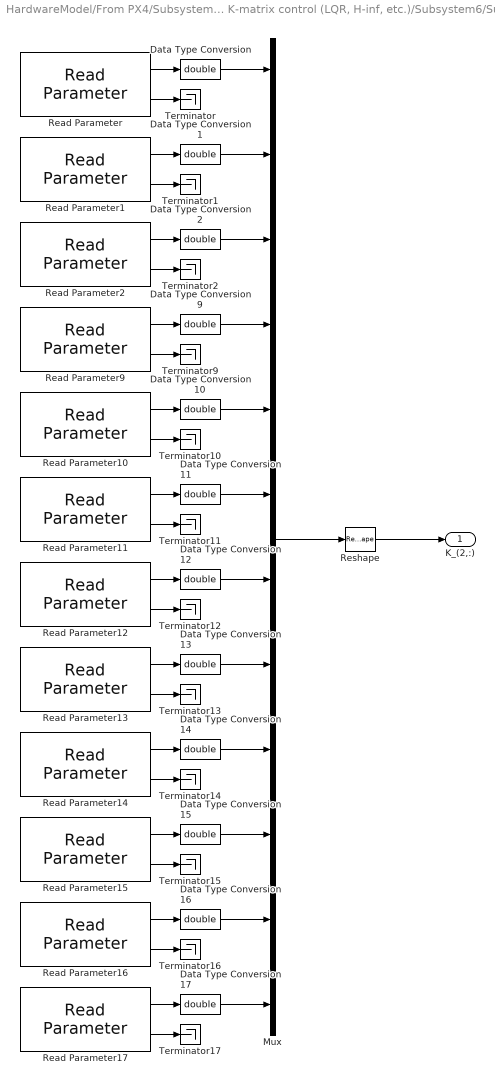
== system HardwareModel/From PX4/Subsystem2/ K-matrix control (LQR, H-inf, etc.)/Subsystem6/Subsystem1 ==
  Data Type Conversion{,1..2,9..17} (12 alike) : DataTypeConversion  OutDataTypeStr=double  SaturateOnIntegerOverflow=off  RndMeth=Floor
  Mux : Mux  Inputs=12
  Read Parameter : px4lib/Read Parameter  ParameterName=SM_K_2_1  DataType=FLOAT  SampleTime=-1
  Read Parameter1 : px4lib/Read Parameter  ParameterName=SM_K_2_2  DataType=FLOAT  SampleTime=-1
  Read Parameter10 : px4lib/Read Parameter  ParameterName=SM_K_2_5  DataType=FLOAT  SampleTime=-1
  Read Parameter11 : px4lib/Read Parameter  ParameterName=SM_K_2_6  DataType=FLOAT  SampleTime=-1
  Read Parameter12 : px4lib/Read Parameter  ParameterName=SM_K_2_7  DataType=FLOAT  SampleTime=-1
  Read Parameter13 : px4lib/Read Parameter  ParameterName=SM_K_2_8  DataType=FLOAT  SampleTime=-1
  Read Parameter14 : px4lib/Read Parameter  ParameterName=SM_K_2_9  DataType=FLOAT  SampleTime=-1
  Read Parameter15 : px4lib/Read Parameter  ParameterName=SM_K_2_10  DataType=FLOAT  SampleTime=-1
  Read Parameter16 : px4lib/Read Parameter  ParameterName=SM_K_2_11  DataType=FLOAT  SampleTime=-1
  Read Parameter17 : px4lib/Read Parameter  ParameterName=SM_K_2_12  DataType=FLOAT  SampleTime=-1
  Read Parameter2 : px4lib/Read Parameter  ParameterName=SM_K_2_3  DataType=FLOAT  SampleTime=-1
  Read Parameter9 : px4lib/Read Parameter  ParameterName=SM_K_2_4  DataType=FLOAT  SampleTime=-1
  Reshape : Reshape  OutputDimensionality=Row vector (2-D)
  Terminator{,1..2,9..17} (12 alike) : Terminator
  K_(2,:) : Outport
  wires:
  Read Parameter15/2 -> Terminator15/1
  Read Parameter9/2 -> Terminator9/1
  Read Parameter17/2 -> Terminator17/1
  Data Type Conversion10/1 -> Mux/5
  Read Parameter12/2 -> Terminator12/1
  Read Parameter14/2 -> Terminator14/1
  Read Parameter14/1 -> Data Type Conversion14/1
  Read Parameter2/2 -> Terminator2/1
  Read Parameter15/1 -> Data Type Conversion15/1
  Data Type Conversion/1 -> Mux/1
  Data Type Conversion11/1 -> Mux/6
  Data Type Conversion17/1 -> Mux/12
  Read Parameter11/1 -> Data Type Conversion11/1
  Data Type Conversion16/1 -> Mux/11
  Read Parameter10/1 -> Data Type Conversion10/1
  Read Parameter17/1 -> Data Type Conversion17/1
  Read Parameter10/2 -> Terminator10/1
  Data Type Conversion15/1 -> Mux/10
  Read Parameter/2 -> Terminator/1
  Data Type Conversion13/1 -> Mux/8
  Read Parameter9/1 -> Data Type Conversion9/1
  Read Parameter/1 -> Data Type Conversion/1
  Read Parameter1/1 -> Data Type Conversion1/1
  Read Parameter13/2 -> Terminator13/1
  Read Parameter1/2 -> Terminator1/1
  Data Type Conversion12/1 -> Mux/7
  Read Parameter11/2 -> Terminator11/1
  Read Parameter2/1 -> Data Type Conversion2/1
  Data Type Conversion2/1 -> Mux/3
  Read Parameter12/1 -> Data Type Conversion12/1
  Read Parameter13/1 -> Data Type Conversion13/1
  Data Type Conversion9/1 -> Mux/4
  Data Type Conversion14/1 -> Mux/9
  Read Parameter16/2 -> Terminator16/1
  Data Type Conversion1/1 -> Mux/2
  Read Parameter16/1 -> Data Type Conversion16/1
  Mux/1 -> Reshape/1
  Reshape/1 -> K_(2,:)/1

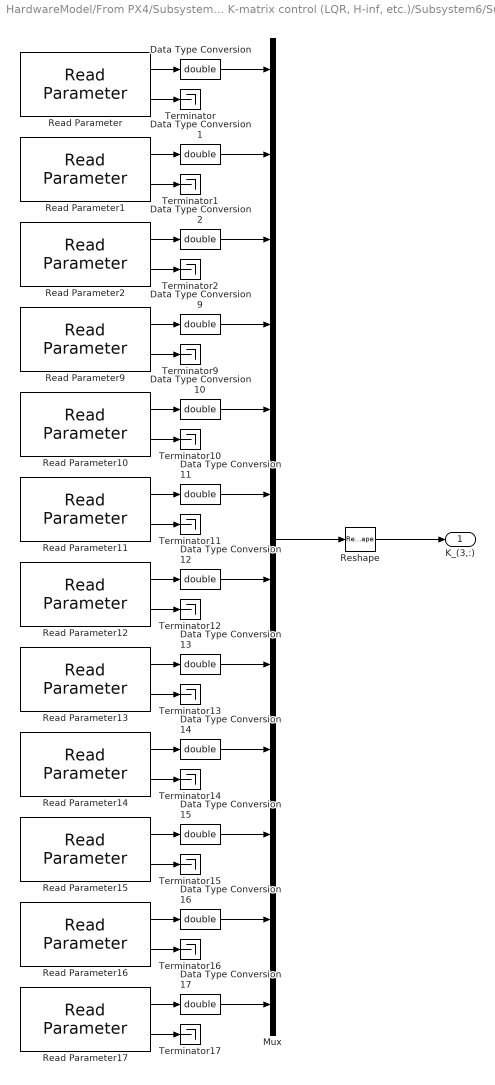
== system HardwareModel/From PX4/Subsystem2/ K-matrix control (LQR, H-inf, etc.)/Subsystem6/Subsystem2 ==
  Data Type Conversion{,1..2,9..17} (12 alike) : DataTypeConversion  OutDataTypeStr=double  SaturateOnIntegerOverflow=off  RndMeth=Floor
  Mux : Mux  Inputs=12
  Read Parameter : px4lib/Read Parameter  ParameterName=SM_K_3_1  DataType=FLOAT  SampleTime=-1
  Read Parameter1 : px4lib/Read Parameter  ParameterName=SM_K_3_2  DataType=FLOAT  SampleTime=-1
  Read Parameter10 : px4lib/Read Parameter  ParameterName=SM_K_3_5  DataType=FLOAT  SampleTime=-1
  Read Parameter11 : px4lib/Read Parameter  ParameterName=SM_K_3_6  DataType=FLOAT  SampleTime=-1
  Read Parameter12 : px4lib/Read Parameter  ParameterName=SM_K_3_7  DataType=FLOAT  SampleTime=-1
  Read Parameter13 : px4lib/Read Parameter  ParameterName=SM_K_3_8  DataType=FLOAT  SampleTime=-1
  Read Parameter14 : px4lib/Read Parameter  ParameterName=SM_K_3_9  DataType=FLOAT  SampleTime=-1
  Read Parameter15 : px4lib/Read Parameter  ParameterName=SM_K_3_10  DataType=FLOAT  SampleTime=-1
  Read Parameter16 : px4lib/Read Parameter  ParameterName=SM_K_3_11  DataType=FLOAT  SampleTime=-1
  Read Parameter17 : px4lib/Read Parameter  ParameterName=SM_K_3_12  DataType=FLOAT  SampleTime=-1
  Read Parameter2 : px4lib/Read Parameter  ParameterName=SM_K_3_3  DataType=FLOAT  SampleTime=-1
  Read Parameter9 : px4lib/Read Parameter  ParameterName=SM_K_3_4  DataType=FLOAT  SampleTime=-1
  Reshape : Reshape  OutputDimensionality=Row vector (2-D)
  Terminator{,1..2,9..17} (12 alike) : Terminator
  K_(3,:) : Outport
  wires:
  Read Parameter15/2 -> Terminator15/1
  Read Parameter9/2 -> Terminator9/1
  Read Parameter17/2 -> Terminator17/1
  Data Type Conversion10/1 -> Mux/5
  Read Parameter12/2 -> Terminator12/1
  Read Parameter14/2 -> Terminator14/1
  Read Parameter14/1 -> Data Type Conversion14/1
  Read Parameter2/2 -> Terminator2/1
  Read Parameter15/1 -> Data Type Conversion15/1
  Data Type Conversion/1 -> Mux/1
  Data Type Conversion11/1 -> Mux/6
  Data Type Conversion17/1 -> Mux/12
  Read Parameter11/1 -> Data Type Conversion11/1
  Data Type Conversion16/1 -> Mux/11
  Read Parameter10/1 -> Data Type Conversion10/1
  Read Parameter17/1 -> Data Type Conversion17/1
  Read Parameter10/2 -> Terminator10/1
  Data Type Conversion15/1 -> Mux/10
  Read Parameter/2 -> Terminator/1
  Data Type Conversion13/1 -> Mux/8
  Read Parameter9/1 -> Data Type Conversion9/1
  Read Parameter/1 -> Data Type Conversion/1
  Read Parameter1/1 -> Data Type Conversion1/1
  Read Parameter13/2 -> Terminator13/1
  Read Parameter1/2 -> Terminator1/1
  Data Type Conversion12/1 -> Mux/7
  Read Parameter11/2 -> Terminator11/1
  Read Parameter2/1 -> Data Type Conversion2/1
  Data Type Conversion2/1 -> Mux/3
  Read Parameter12/1 -> Data Type Conversion12/1
  Read Parameter13/1 -> Data Type Conversion13/1
  Data Type Conversion9/1 -> Mux/4
  Data Type Conversion14/1 -> Mux/9
  Read Parameter16/2 -> Terminator16/1
  Data Type Conversion1/1 -> Mux/2
  Read Parameter16/1 -> Data Type Conversion16/1
  Mux/1 -> Reshape/1
  Reshape/1 -> K_(3,:)/1

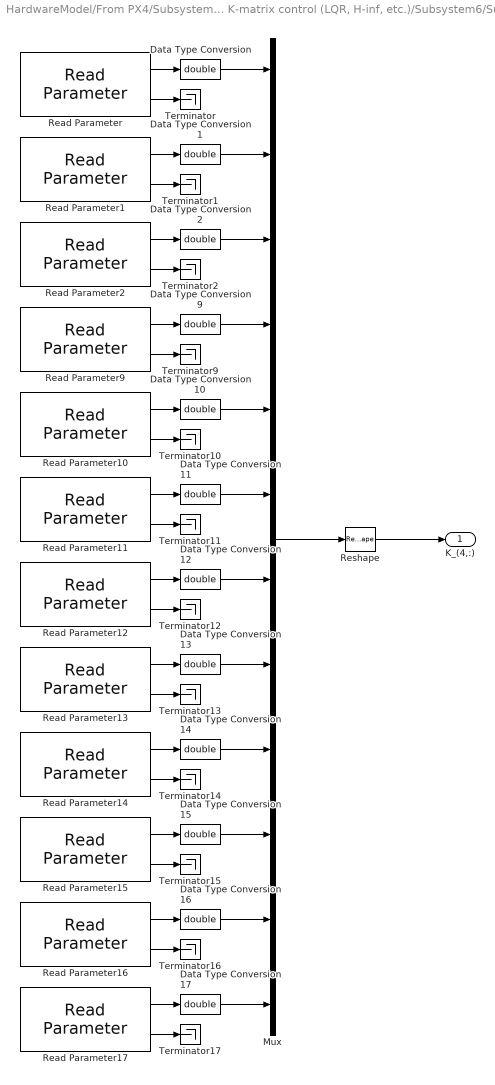
== system HardwareModel/From PX4/Subsystem2/ K-matrix control (LQR, H-inf, etc.)/Subsystem6/Subsystem3 ==
  Data Type Conversion{,1..2,9..17} (12 alike) : DataTypeConversion  OutDataTypeStr=double  SaturateOnIntegerOverflow=off  RndMeth=Floor
  Mux : Mux  Inputs=12
  Read Parameter : px4lib/Read Parameter  ParameterName=SM_K_4_1  DataType=FLOAT  SampleTime=-1
  Read Parameter1 : px4lib/Read Parameter  ParameterName=SM_K_4_2  DataType=FLOAT  SampleTime=-1
  Read Parameter10 : px4lib/Read Parameter  ParameterName=SM_K_4_5  DataType=FLOAT  SampleTime=-1
  Read Parameter11 : px4lib/Read Parameter  ParameterName=SM_K_4_6  DataType=FLOAT  SampleTime=-1
  Read Parameter12 : px4lib/Read Parameter  ParameterName=SM_K_4_7  DataType=FLOAT  SampleTime=-1
  Read Parameter13 : px4lib/Read Parameter  ParameterName=SM_K_4_8  DataType=FLOAT  SampleTime=-1
  Read Parameter14 : px4lib/Read Parameter  ParameterName=SM_K_4_9  DataType=FLOAT  SampleTime=-1
  Read Parameter15 : px4lib/Read Parameter  ParameterName=SM_K_4_10  DataType=FLOAT  SampleTime=-1
  Read Parameter16 : px4lib/Read Parameter  ParameterName=SM_K_4_11  DataType=FLOAT  SampleTime=-1
  Read Parameter17 : px4lib/Read Parameter  ParameterName=SM_K_4_12  DataType=FLOAT  SampleTime=-1
  Read Parameter2 : px4lib/Read Parameter  ParameterName=SM_K_4_3  DataType=FLOAT  SampleTime=-1
  Read Parameter9 : px4lib/Read Parameter  ParameterName=SM_K_4_4  DataType=FLOAT  SampleTime=-1
  Reshape : Reshape  OutputDimensionality=Row vector (2-D)
  Terminator{,1..2,9..17} (12 alike) : Terminator
  K_(4,:) : Outport
  wires:
  Read Parameter15/2 -> Terminator15/1
  Read Parameter9/2 -> Terminator9/1
  Read Parameter17/2 -> Terminator17/1
  Data Type Conversion10/1 -> Mux/5
  Read Parameter12/2 -> Terminator12/1
  Read Parameter14/2 -> Terminator14/1
  Read Parameter14/1 -> Data Type Conversion14/1
  Read Parameter2/2 -> Terminator2/1
  Read Parameter15/1 -> Data Type Conversion15/1
  Data Type Conversion/1 -> Mux/1
  Data Type Conversion11/1 -> Mux/6
  Data Type Conversion17/1 -> Mux/12
  Read Parameter11/1 -> Data Type Conversion11/1
  Data Type Conversion16/1 -> Mux/11
  Read Parameter10/1 -> Data Type Conversion10/1
  Read Parameter17/1 -> Data Type Conversion17/1
  Read Parameter10/2 -> Terminator10/1
  Data Type Conversion15/1 -> Mux/10
  Read Parameter/2 -> Terminator/1
  Data Type Conversion13/1 -> Mux/8
  Read Parameter9/1 -> Data Type Conversion9/1
  Read Parameter/1 -> Data Type Conversion/1
  Read Parameter1/1 -> Data Type Conversion1/1
  Read Parameter13/2 -> Terminator13/1
  Read Parameter1/2 -> Terminator1/1
  Data Type Conversion12/1 -> Mux/7
  Read Parameter11/2 -> Terminator11/1
  Read Parameter2/1 -> Data Type Conversion2/1
  Data Type Conversion2/1 -> Mux/3
  Read Parameter12/1 -> Data Type Conversion12/1
  Read Parameter13/1 -> Data Type Conversion13/1
  Data Type Conversion9/1 -> Mux/4
  Data Type Conversion14/1 -> Mux/9
  Read Parameter16/2 -> Terminator16/1
  Data Type Conversion1/1 -> Mux/2
  Read Parameter16/1 -> Data Type Conversion16/1
  Mux/1 -> Reshape/1
  Reshape/1 -> K_(4,:)/1

== system HardwareModel/From PX4/Subsystem5/Subsystem/Subsystem1/Disabled ==
  Constant : Constant  Value=0
  Constant1 : Constant  Value=0
  Constant19 : Constant  Value=flight_mode.position_hold
  Constant2 : Constant  Value=0
  Constant3 : Constant  Value=-1
  Constant4 : Constant  Value=false
  roll_stick : Outport
  pitch_stick : Outport  Port=2
  yaw_stick : Outport  Port=3
  Throttle_stick : Outport  Port=4
  FLIGHT_MODE : Outport  Port=5
  ARMED : Outport  Port=6
  wires:
  Constant3/1 -> Throttle_stick/1  "Throttle_stick"
  Constant1/1 -> pitch_stick/1  "pitch_stick"
  Constant/1 -> roll_stick/1  "roll_stick"
  Constant2/1 -> yaw_stick/1  "yaw_stick"
  Constant19/1 -> FLIGHT_MODE/1  "FLIGHT_MODE"
  Constant4/1 -> ARMED/1  "ARMED"

== system HardwareModel/From PX4/Subsystem5/Subsystem/Subsystem1/Joytick ==
  Constant14 : Constant  Value=joystick.sticks.cal.min
  Constant15 : Constant  Value=joystick.sticks.cal.max
  Constant16 : Constant  Value=joystick.sticks.n
  Constant17 : Constant  Value=joystick.sticks.cal.vals
  Constant4 : Constant  Value=true
  Joystick Input : vrlib/Joystick Input  joyid=1  adjustports=on  forcefeed=off
  MATLAB Function : MATLAB Function  TreatAsAtomicUnit=on
  Terminator : Terminator
  roll_stick : Outport
  pitch_stick : Outport  Port=2
  yaw_stick : Outport  Port=3
  Throttle_stick : Outport  Port=4
  FLIGHT_MODE : Outport  Port=5
  ARMED : Outport  Port=6
  wires:
  Constant15/1 -> MATLAB Function/5(max)
  Constant14/1 -> MATLAB Function/4(min)
  MATLAB Function/4(throttle_stick) -> Throttle_stick/1  "Throttle_stick"
  Constant16/1 -> MATLAB Function/3(n)
  Constant17/1 -> MATLAB Function/6(vals)
  Joystick Input/1 -> MATLAB Function/1(sticks)
  MATLAB Function/2(pitch_stick) -> pitch_stick/1  "pitch_stick"
  Joystick Input/2 -> MATLAB Function/2(buttons)
  ? -> Terminator/1
  MATLAB Function/1(roll_stick) -> roll_stick/1  "roll_stick"
  MATLAB Function/3(yaw_stick) -> yaw_stick/1  "yaw_stick"
  MATLAB Function/5(FLIGHT_MODE) -> FLIGHT_MODE/1  "FLIGHT_MODE"
  Constant4/1 -> ARMED/1  "ARMED"

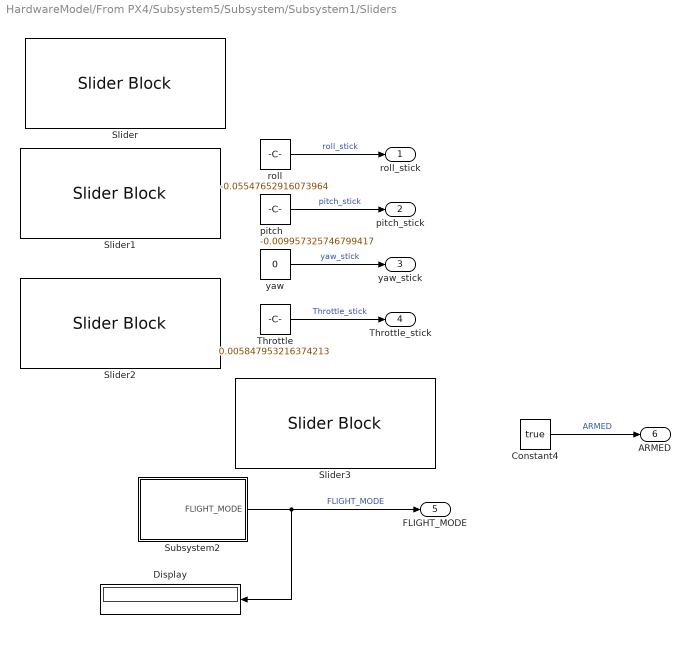
== system HardwareModel/From PX4/Subsystem5/Subsystem/Subsystem1/Sliders ==
  Constant4 : Constant  Value=true
  Display : Display
  Slider{,1..3} (4 alike) : SliderBlock  ScaleMin=-1  ScaleMax=1
  Subsystem2 : Subsystem
  Throttle : Constant  Value=0.005847953216374213
  pitch : Constant  Value=-0.009957325746799417
  roll : Constant  Value=-0.05547652916073964
  yaw : Constant  Value=0
  roll_stick : Outport
  pitch_stick : Outport  Port=2
  yaw_stick : Outport  Port=3
  Throttle_stick : Outport  Port=4
  FLIGHT_MODE : Outport  Port=5
  ARMED : Outport  Port=6
  wires:
  roll/1 -> roll_stick/1  "roll_stick"
  yaw/1 -> yaw_stick/1  "yaw_stick"
  pitch/1 -> pitch_stick/1  "pitch_stick"
  Throttle/1 -> Throttle_stick/1  "Throttle_stick"
  Subsystem2/1(FLIGHT_MODE) -> FLIGHT_MODE/1, Display/1  "FLIGHT_MODE"
  Constant4/1 -> ARMED/1  "ARMED"

== system HardwareModel/From PX4/Subsystem5/Subsystem/Subsystem1/Sliders/Subsystem2 ==
  Constant19 : Constant  Value=FLIGHT_MODE
  Constant3 : Constant  Value=flight_mode.autonomous
  Equal : RelationalOperator  Operator===  OutDataTypeStr=boolean  RndMeth=Simplest  InputSameDT=off
  If : If  IfExpression=u1
  If Action Subsystem : Subsystem  TreatAsAtomicUnit=on
  If Action Subsystem1 : Subsystem  TreatAsAtomicUnit=on
  Merge : Merge
  FLIGHT_MODE : Outport
  wires:
  If/1 -> If Action Subsystem/Action
  If Action Subsystem1/1(Out1) -> Merge/2
  Merge/1 -> FLIGHT_MODE/1
  Constant19/1 -> If Action Subsystem1/1(In1), Equal/1  "FLIGHT_MODE"
  Constant3/1 -> Equal/2
  Equal/1 -> If/1
  If/2 -> If Action Subsystem1/Action
  If Action Subsystem/1(Out1) -> Merge/1

== system HardwareModel/From PX4/Subsystem5/Subsystem/Subsystem1/Sliders/Subsystem2/If Action Subsystem ==
  Action Port : ActionPort
  Clock : Clock
  Constant : Constant  Value=flight_mode.autonomous
  Constant1 : Constant  Value=flight_mode.position_hold
  Constant2 : Constant  Value=wait_time_s
  GreaterThan : RelationalOperator  Operator=<  OutDataTypeStr=boolean  RndMeth=Simplest  InputSameDT=off
  Multiport Switch1 : MultiPortSwitch  DataPortOrder=Zero-based contiguous  Inputs=2  DiagnosticForDefault=None  zeroidx=on  SaturateOnIntegerOverflow=off  InputSameDT=off
  Out1 : Outport
  wires:
  Constant2/1 -> GreaterThan/2
  Constant1/1 -> Multiport Switch1/3
  GreaterThan/1 -> Multiport Switch1/1
  Constant/1 -> Multiport Switch1/2
  Multiport Switch1/1 -> Out1/1
  Clock/1 -> GreaterThan/1

== system HardwareModel/From PX4/Subsystem5/Subsystem/Subsystem1/Sliders/Subsystem2/If Action Subsystem1 ==
  In1 : Inport
  Action Port : ActionPort
  Out1 : Outport
  wires:
  In1/1 -> Out1/1

== matlab function HardwareModel/From PX4/Subsystem5/Subsystem/Subsystem1/Joytick/MATLAB Function ==
  data: sticks input; roll_stick output; buttons input; n input; min input; max input; pitch_stick output; yaw_stick output; throttle_stick output; vals input; FLIGHT_MODE output
function [roll_stick, pitch_stick, yaw_stick, throttle_stick, FLIGHT_MODE] = fcn(sticks, buttons, n, min, max, vals)
joystick.sticks.raw = sticks;
joystick.buttons.raw = buttons;
joystick.sticks.n = n;
joystick.sticks.cal.min = min;
joystick.sticks.cal.max = max;
joystick.sticks.cal.vals = vals;

ROLL_STICK = 1;
PITCH_STICK = 2;
THROTTLE_STICK = 3;
YAW_STICK = 5;
AUX1_STICK = 4;

StickMap = [...
    ROLL_STICK
    PITCH_STICK
    YAW_STICK
    THROTTLE_STICK
    AUX1_STICK];

ROLL_STICK_POL = 1;
PITCH_STICK_POL = -1;
THROTTLE_STICK_POL = -1;
YAW_STICK_POL = 1;
AUX1_STICK_POL = 1;

StickPol = [...
    ROLL_STICK_POL
    PITCH_STICK_POL
    YAW_STICK_POL
    THROTTLE_STICK_POL
    AUX1_STICK_POL];

% tol = 1E-12;
deadzone_RPY = 0.05; %sticks are not perfectly centered 
deadzone_Z = 0.05;
joystick = lib.joystick.apply_cal(joystick);
mapped_sticks = joystick.sticks.cal.vals(StickMap);
mapped_sticks = mapped_sticks(:).*StickPol(:);
roll_stick = lib.math.apply_deadzone(mapped_sticks(1),deadzone_RPY,0);
pitch_stick = lib.math.apply_deadzone(mapped_sticks(2),deadzone_RPY,0);
yaw_stick = lib.math.apply_deadzone(mapped_sticks(3),deadzone_RPY,0);
throttle_stick = lib.math.apply_deadzone(mapped_sticks(4),deadzone_Z,0);

button_case = 0;
flight_mode_buttons = buttons(4:5);
if flight_mode_buttons(1) == 0 && flight_mode_buttons(2) == 0
    button_case = 0;
elseif flight_mode_buttons(1) == 1
    button_case = 1;
elseif flight_mode_buttons(2) == 1
    button_case = 2;
end


switch button_case
    case 2
        FLIGHT_MODE = flight_mode.autonomous;
    case 1
        FLIGHT_MODE = flight_mode.attitude_control;
        % FLIGHT_MODE = flight_mode.position_control;
    case 0
        % FLIGHT_MODE = flight_mode.attitude_control;
        FLIGHT_MODE = flight_mode.position_control;
    otherwise 
        FLIGHT_MODE = flight_mode.position_hold;
end

end
